simulink model "model2"  (R2015a)
settings: Solver=ode3  StartTime=0.0  StopTime=10.0  FixedStep=0.001  RelTol=1e-3
values from neighbouring files (symbols this model uses):
  th0 = 1    [starter2.m]
  thd0 = 0    [starter2.m]
  x0 = 1    [starter2.m]
  xd0 = 0    [starter2.m]
  z0 = 1    [starter2.m]
  zd0 = 0    [starter2.m]
settings Model: Creator=zanez  LastModifiedBy=Subodh

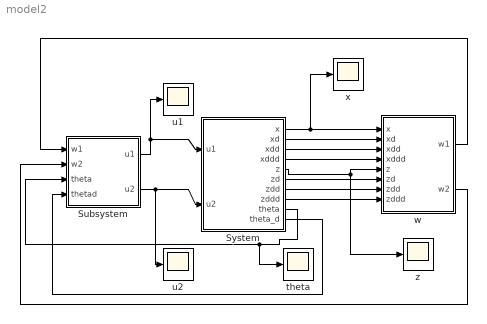
== system model2 ==
  Subsystem : Subsystem
  System : Subsystem
  theta : Scope
      settings: TimeRange=auto  MaxDataPoints=5000  SaveName=theta  YMin=-0.86685  YMax=2.52181  SampleTime=-1  DataFormat=Array
  u1 : Scope
      settings: TimeRange=auto  MaxDataPoints=5000  SaveName=u1  YMin=0.22219  YMax=4.19947  SampleTime=-1  DataFormat=Array
  u2 : Scope
      settings: TimeRange=auto  MaxDataPoints=5000  SaveName=u2  YMin=-522.12281  YMax=877.33327  SampleTime=-1  DataFormat=Array
  w : Subsystem
  x : Scope
      settings: TimeRange=auto  MaxDataPoints=5000  SaveName=x  YMin=-0.125  YMax=1.125  SampleTime=-1  DataFormat=Array
  z : Scope
      settings: TimeRange=auto  MaxDataPoints=5000  SaveName=z  YMin=-0.125  YMax=1.125  SampleTime=-1  DataFormat=Array
  wires:
  System/9(theta) -> theta/1, Subsystem/3(theta)
  Subsystem/2(u2) -> System/2(u2), u2/1
  Subsystem/1(u1) -> u1/1, System/1(u1)
  w/1(w1) -> Subsystem/1(w1)
  w/2(w2) -> Subsystem/2(w2)
  System/10(theta_d) -> Subsystem/4(thetad)
  System/1(x) -> x/1, w/1(x)
  System/2(xd) -> w/2(xd)
  System/3(xdd) -> w/3(xdd)
  System/4(xddd) -> w/4(xddd)
  System/5(z) -> w/5(z), z/1
  System/6(zd) -> w/6(zd)
  System/7(zdd) -> w/7(zdd)
  System/8(zddd) -> w/8(zddd)

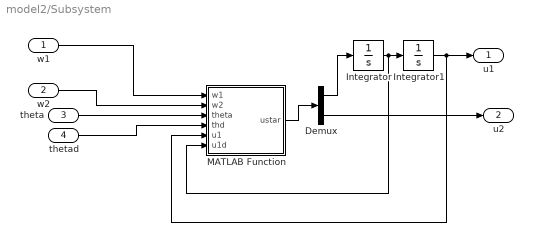
== system model2/Subsystem ==
  w1 : Inport
  w2 : Inport  Port=2
  theta : Inport  Port=3
  thetad : Inport  Port=4
  Demux : Demux  Outputs=2
  Integrator : Integrator
  Integrator1 : Integrator  InitialCondition=1
  MATLAB Function : MATLAB Function  TreatAsAtomicUnit=on
      settings: PermitHierarchicalResolution=ParametersOnly
  u1 : Outport
  u2 : Outport  Port=2
  wires:
  theta/1 -> MATLAB Function/3(theta)
  Demux/2 -> u2/1
  MATLAB Function/1(ustar) -> Demux/1
  w1/1 -> MATLAB Function/1(w1)
  w2/1 -> MATLAB Function/2(w2)
  Demux/1 -> Integrator/1
  Integrator/1 -> MATLAB Function/6(u1d), Integrator1/1
  Integrator1/1 -> u1/1, MATLAB Function/5(u1)
  thetad/1 -> MATLAB Function/4(thd)

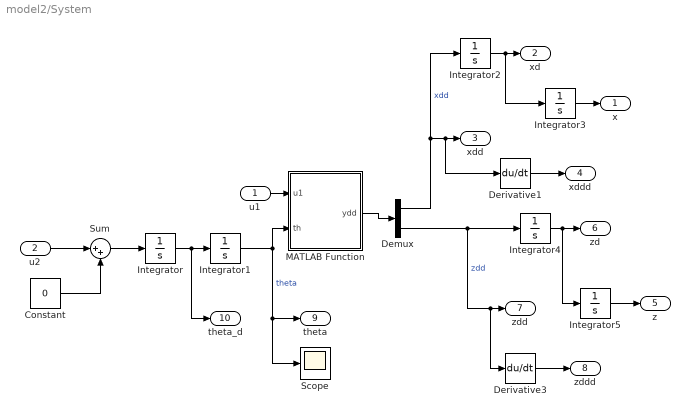
== system model2/System ==
  u1 : Inport
  u2 : Inport  Port=2
  Constant : Constant  Value=0
  Demux : Demux  Outputs=2
  Derivative1 : Derivative
  Derivative3 : Derivative
  Integrator : Integrator  InitialCondition=thd0
  Integrator1 : Integrator  InitialCondition=th0
  Integrator2 : Integrator  InitialCondition=xd0
  Integrator3 : Integrator  InitialCondition=x0
  Integrator4 : Integrator  InitialCondition=zd0
  Integrator5 : Integrator  InitialCondition=z0
  MATLAB Function : MATLAB Function  TreatAsAtomicUnit=on
      settings: PermitHierarchicalResolution=ParametersOnly
  Scope : Scope
      settings: TimeRange=auto  LimitDataPoints=on  MaxDataPoints=5000  SaveToWorkspace=off  SaveName=ScopeData  YMin=-10  YMax=10  SampleTime=-1  DataFormat=Array
  Sum : Sum  Inputs=|++
  x : Outport
  xd : Outport  Port=2
  xdd : Outport  Port=3
  xddd : Outport  Port=4
  z : Outport  Port=5
  zd : Outport  Port=6
  zdd : Outport  Port=7
  zddd : Outport  Port=8
  theta : Outport  Port=9
  theta_d : Outport  Port=10
  wires:
  Integrator2/1 -> Integrator3/1, xd/1
  Demux/1 -> Derivative1/1, xdd/1, Integrator2/1  "xdd"
  Integrator3/1 -> x/1
  Integrator4/1 -> Integrator5/1, zd/1
  Integrator5/1 -> z/1
  MATLAB Function/1(ydd) -> Demux/1
  Demux/2 -> zdd/1, Derivative3/1, Integrator4/1  "zdd"
  u1/1 -> MATLAB Function/1(u1)
  Derivative1/1 -> xddd/1
  Derivative3/1 -> zddd/1
  u2/1 -> Sum/1
  Constant/1 -> Sum/2
  Integrator/1 -> Integrator1/1, theta_d/1
  Sum/1 -> Integrator/1
  Integrator1/1 -> MATLAB Function/2(th), Scope/1, theta/1  "theta"

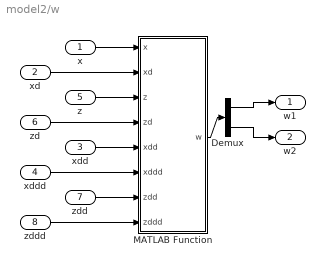
== system model2/w ==
  x : Inport
  xd : Inport  Port=2
  xdd : Inport  Port=3
  xddd : Inport  Port=4
  z : Inport  Port=5
  zd : Inport  Port=6
  zdd : Inport  Port=7
  zddd : Inport  Port=8
  Demux : Demux  Outputs=2
  MATLAB Function : MATLAB Function  TreatAsAtomicUnit=on
      settings: PermitHierarchicalResolution=ParametersOnly
  w1 : Outport
  w2 : Outport  Port=2
  wires:
  xd/1 -> MATLAB Function/2(xd)
  x/1 -> MATLAB Function/1(x)
  zd/1 -> MATLAB Function/4(zd)
  z/1 -> MATLAB Function/3(z)
  MATLAB Function/1(w) -> Demux/1
  Demux/1 -> w1/1
  Demux/2 -> w2/1
  xdd/1 -> MATLAB Function/5(xdd)
  zdd/1 -> MATLAB Function/7(zdd)
  zddd/1 -> MATLAB Function/8(zddd)
  xddd/1 -> MATLAB Function/6(xddd)

== matlab function model2/System/MATLAB Function ==
  data: u1 input; ydd output; th input
function ydd = fcn(u1, th)
%#codegen
xdd = -u1*sin(th);
zdd = u1*cos(th)-1;
ydd = [xdd;zdd];

== matlab function model2/Subsystem/MATLAB Function ==
  data: ustar output; w1 input; w2 input; theta input; thd input; u1 input; u1d input
function ustar = fcn(w1,w2, theta, thd, u1,u1d)
%#codegen
th = theta;
bstar = [    -sin(th),     -u1*cos(th); cos(th), -u1*sin(th)];
bstarI = [    -sin(th),     cos(th); -cos(th)/u1, -sin(th)/u1];
w1ma = w1 + 2*u1d*cos(th)*thd-u1*sin(th)*thd^2;
w2ma = w2 + 2*u1d*sin(th)*thd+u1*cos(th)*thd^2;

ustar = bstarI*[w1ma;w2ma];

== matlab function model2/w/MATLAB Function ==
  data: x input; xd input; z input; w output; zd input; xdd input; xddd input; zdd input; zddd input
function w = fcn(x,xd,z, zd, xdd, xddd, zdd, zddd)
%#codegen
s0 = 5;
k11 = 4*s0; k12 = 6*s0^2; k13 = 4*s0^3; k14 = s0^4;
k21 = 4*s0; k22 = 6*s0^2; k23 = 4*s0^3; k24 = s0^4;
w1 = -k11*xddd-k12*xdd-k13*xd-k14*x;
w2 = -k21*zddd-k22*zdd-k23*zd-k24*z;
w = [w1;w2];
